simulink model "m_goldoozian"  (R2020a)
settings: Solver=FixedStepAuto  StartTime=0.0  StopTime=100  FixedStep=0.001  RelTol=1e-3
undefined symbols (not defined in the file): alpha, b_h, Ca, delta_h, DeltaV, gamma, H0, k1, k2, P_o, Rco, RR, tau, TV, V_h
settings Model: Creator=sebastian  LastModifiedBy=sebastian

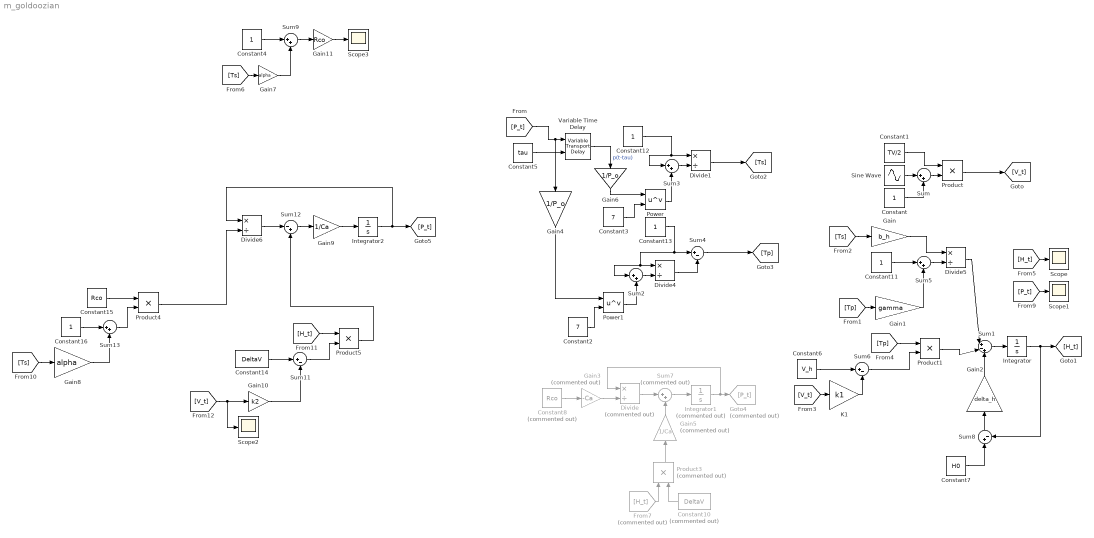
== system m_goldoozian ==
  Constant{,4,11..13,16} (6 alike) : Constant
  Constant1 : Constant  Value=TV/2
  Constant10 : Constant  Commented=on  Value=DeltaV
  Constant14 : Constant  Value=DeltaV
  Constant15 : Constant  Value=Rco
  Constant2 : Constant  Value=7
  Constant3 : Constant  Value=7
  Constant5 : Constant  Value=tau
  Constant6 : Constant  Value=V_h
  Constant7 : Constant  Value=H0
  Constant8 : Constant  Commented=on  Value=Rco
  Divide : Product  Commented=on  Inputs=*/
  Divide{1,4..6} (4 alike) : Product  Inputs=*/
  From7 : From  Commented=on  GotoTag=H_t
  Gain : Gain  Gain=b_h
  Gain1 : Gain  Gain=gamma
  Gain10 : Gain  Gain=k2
  Gain11 : Gain  Gain=Rco
  Gain2 : Gain  Gain=delta_h
  Gain3 : Gain  Commented=on  Gain=-Ca
  Gain4 : Gain  Gain=1/P_o
  Gain5 : Gain  Commented=on  Gain=1/Ca
  Gain6 : Gain  Gain=1/P_o
  Gain7 : Gain  Gain=alpha
  Gain8 : Gain  Gain=alpha
  Gain9 : Gain  Gain=1/Ca
  Goto4 : Goto  Commented=on  GotoTag=P_t
  Integrator : Integrator
  Integrator1 : Integrator  Commented=on
  Integrator2 : Integrator  InitialCondition=0.1
  K1 : Gain  Gain=k1
  Power : Math  Operator=pow  SaturateOnIntegerOverflow=on
  Power1 : Math  Operator=pow  SaturateOnIntegerOverflow=on
  Product{,1,4..5} (4 alike) : Product
  Product3 : Product  Commented=on
  Scope{,1..3} (4 alike) : Scope
  Sine Wave : Sin  Frequency=2*pi*RR  Phase=-pi/2  SampleTime=0
  Sum{,2..3,5,9,13} (6 alike) : Sum  Inputs=|++
  Sum1 : Sum  Inputs=|+-+
  Sum{4,6,8,11} (4 alike) : Sum  Inputs=|+-
  Sum12 : Sum  Inputs=|-+
  Sum7 : Sum  Commented=on  Inputs=|++
  Variable Time Delay : VariableTransportDelay  MaximumDelay=10
  wires:
  Sine Wave/1 -> Sum/1
  Constant/1 -> Sum/2
  Sum/1 -> Product/2
  Constant1/1 -> Product/1
  Product/1 -> [V_t]
  Integrator/1 -> [H_t], Sum8/2
  Sum1/1 -> Integrator/1
  Constant5/1 -> Variable Time Delay/2
  Variable Time Delay/1 -> Gain6/1  "p(t-tau)"
  Sum3/1 -> Divide1/2
  Divide1/1 -> [Ts]
  Sum2/1 -> Divide4/2
  Divide4/1 -> Sum4/2
  Sum4/1 -> [Tp]
  [Ts] -> Gain/1
  Gain/1 -> Divide5/1
  [Tp] -> Gain1/1
  Gain1/1 -> Sum5/2
  Sum5/1 -> Divide5/2
  Divide5/1 -> Sum1/1
  [Tp] -> Product1/1
  [V_t] -> K1/1
  K1/1 -> Sum6/2
  Constant6/1 -> Sum6/1
  Sum6/1 -> Product1/2
  Product1/1 -> Sum1/2
  Constant7/1 -> Sum8/1
  Sum8/1 -> Gain2/1
  Gain2/1 -> Sum1/3
  [H_t] -> Scope/1
  Sum7/1 -> Integrator1/1
  Integrator1/1 -> Goto4/1, Divide/1
  Divide/1 -> Sum7/1
  Constant8/1 -> Gain3/1
  Gain3/1 -> Divide/2
  Gain5/1 -> Sum7/2
  From7/1 -> Product3/1
  Product3/1 -> Gain5/1
  Constant11/1 -> Sum5/1
  Constant12/1 -> Divide1/1, Sum3/1
  Constant13/1 -> Divide4/1, Sum2/1, Sum4/1
  Constant3/1 -> Power/2
  Power/1 -> Sum3/2
  Constant2/1 -> Power1/2
  [P_t] -> Variable Time Delay/1, Gain4/1
  Power1/1 -> Sum2/2
  [P_t] -> Scope1/1
  Sum11/1 -> Product5/2
  Constant15/1 -> Product4/1
  Constant16/1 -> Sum13/1
  Constant14/1 -> Sum11/1
  Sum13/1 -> Product4/2
  Product5/1 -> Sum12/2
  [H_t] -> Product5/1
  Integrator2/1 -> Divide6/1, [P_t]
  Gain8/1 -> Sum13/2
  [Ts] -> Gain8/1
  Divide6/1 -> Sum12/1
  Gain10/1 -> Sum11/2
  Product4/1 -> Divide6/2
  [V_t] -> Scope2/1, Gain10/1
  Sum12/1 -> Gain9/1
  Constant10/1 -> Product3/2
  Gain4/1 -> Power1/1
  Gain6/1 -> Power/1
  Gain9/1 -> Integrator2/1
  Constant4/1 -> Sum9/1
  [Ts] -> Gain7/1
  Gain7/1 -> Sum9/2
  Sum9/1 -> Gain11/1
  Gain11/1 -> Scope3/1
